simulink model "dec_consensus_dead"  (R2022b)
settings: Solver=FixedStepAuto  StartTime=0.0  StopTime=tf  FixedStep=dt  RelTol=1e-3
values from neighbouring files (symbols this model uses):
  A_an_n2 = ss_An.A    [squared_formation_dec.m]
  A_an_n3 = ss_An.A    [squared_formation_dec.m]
  A_an_n4 = ss_An.A    [squared_formation_dec.m]
  A_an_n6 = ss_An.A    [squared_formation_dec.m]
  alpha = binvar(nt,nr)    [main_red_based_TA.m]    (also in motivating_ex_four.m = 25; old_red_based_TA.m = binvar(nt*nr,1); red_consensus.m = 50; red_consensus_2D.m = 50)
  B = eye(n)    [red_consensus.m]    (also in red_consensus_2D.m = eye(2*n); rendez_vous.m = eye(2*n_t3); squared_formation.m = eye(2*n_t2); squared_formation_dec.m = eye(2*n_t2))
  B_an_n2 = ss_An.B    [squared_formation_dec.m]
  B_an_n3 = ss_An.B    [squared_formation_dec.m]
  B_an_n4 = ss_An.B    [squared_formation_dec.m]
  B_an_n6 = ss_An.B    [squared_formation_dec.m]
  C_an_n2 = ss_An.C    [squared_formation_dec.m]
  C_an_n3 = ss_An.C    [squared_formation_dec.m]
  C_an_n4 = ss_An.C    [squared_formation_dec.m]
  C_an_n6 = ss_An.C    [squared_formation_dec.m]
  C_n2 = blkdiag(L_n2,L_n2)    [squared_formation_dec.m]
  C_n3 = blkdiag(L_n3,L_n3)    [squared_formation_dec.m]
  C_n4 = blkdiag(L_n4,L_n4)    [squared_formation_dec.m]
  C_n6 = blkdiag(L_n6,L_n6)    [squared_formation_dec.m]
  C_opt = 1    [motivating_ex_four.m]    (also in red_consensus.m; red_consensus_2D.m = eye(2); rendez_vous.m = eye(2); squared_formation.m = eye(2))
  D_an_n2 = ss_An.D    [squared_formation_dec.m]
  D_an_n3 = ss_An.D    [squared_formation_dec.m]
  D_an_n4 = ss_An.D    [squared_formation_dec.m]
  D_an_n6 = ss_An.D    [squared_formation_dec.m]
  delta_n2 = [delta_x_t2(Idx2);delta_y_t2(Idx2)]    [squared_formation_dec.m]
  delta_n3 = [delta_x_t2(Idx3);delta_y_t2(Idx3)]    [squared_formation_dec.m]
  delta_n4 = [delta_x_t2(Idx4);delta_y_t2(Idx4)]    [squared_formation_dec.m]
  delta_n6 = [delta_x_t2(Idx6);delta_y_t2(Idx6)]    [squared_formation_dec.m]
  f = 0.2    [consensus.m]    (also in consensus_sat.m; red_consensus.m = 1; red_consensus_2D.m; rendez_vous.m)
  sig_vec = ones(num,1)    [rendez_vous.m]    (also in squared_formation.m; squared_formation_dec.m; triangular_formation.m)
  th = 0.05    [motivating_ex_four.m]    (also in red_consensus.m; red_consensus_2D.m; triangular_formation.m)
  u_max_n2 = [u_max1;u_max2;u_max3]    [motivating_ex_four.m]    (also in squared_formation_dec.m = [u_max_x(idx_n2);u_max_y(idx_n2)])
  u_max_n3 = [u_max2;u_max3;u_max4]    [motivating_ex_four.m]    (also in squared_formation_dec.m = [u_max_x(idx_n3);u_max_y(idx_n3)])
  u_max_n4 = [u_max3;u_max4]    [motivating_ex_four.m]    (also in squared_formation_dec.m = [u_max_x(idx_n4);u_max_y(idx_n4)])
  u_max_n6 = [u_max_x(idx_n6);u_max_y(idx_n6)]    [squared_formation_dec.m]
  W_an0_n2 = dcgain(W_an)    [squared_formation_dec.m]
  W_an0_n3 = dcgain(W_an)    [squared_formation_dec.m]
  W_an0_n4 = dcgain(W_an)    [squared_formation_dec.m]
  W_an0_n6 = dcgain(W_an)    [squared_formation_dec.m]
  x0_n2 = x0_cc2(Idx2)    [squared_formation_dec.m]
  x0_n3 = x0_cc2(Idx3)    [squared_formation_dec.m]
  x0_n4 = x0_cc2(Idx4)    [squared_formation_dec.m]
  x0_n6 = x0_cc2(Idx6)    [squared_formation_dec.m]
  x_an0 = zeros(max(size(A_an)),1)    [red_consensus.m]    (also in red_consensus_2D.m; rendez_vous.m; squared_formation.m; squared_formation_dec.m = zeros(max(size(A_an_n2)),1))
  x_opt0 = 0    [red_consensus.m]    (also in red_consensus_2D.m = zeros(2,1); rendez_vous.m = zeros(2,1); squared_formation.m = zeros(2,1); squared_formation_dec.m = zeros(2,1))
  y0_n2 = y0_cc2(Idx2)    [squared_formation_dec.m]
  y0_n3 = y0_cc2(Idx3)    [squared_formation_dec.m]
  y0_n4 = y0_cc2(Idx4)    [squared_formation_dec.m]
  y0_n6 = y0_cc2(Idx6)    [squared_formation_dec.m]
settings Model: Creator=lorenzo  LastModifiedBy=lorenzo
settings SolverCC: ZeroCrossControl=DisableAll
settings OptimizationCC: ReuseModelBlockBuffer=on
settings DebuggingCC: IgnoredZcDiagnostic=none

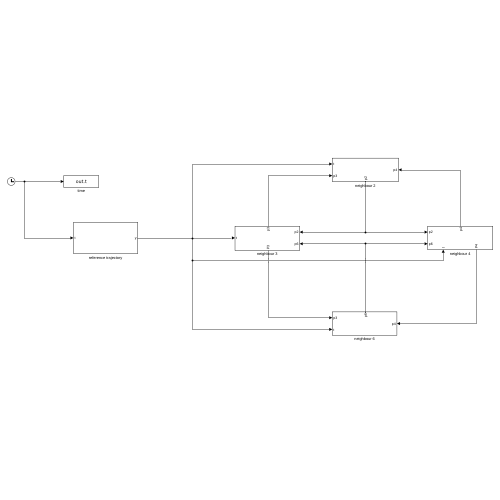
[thumbnail: Simulink's stored preview of the top-level diagram]
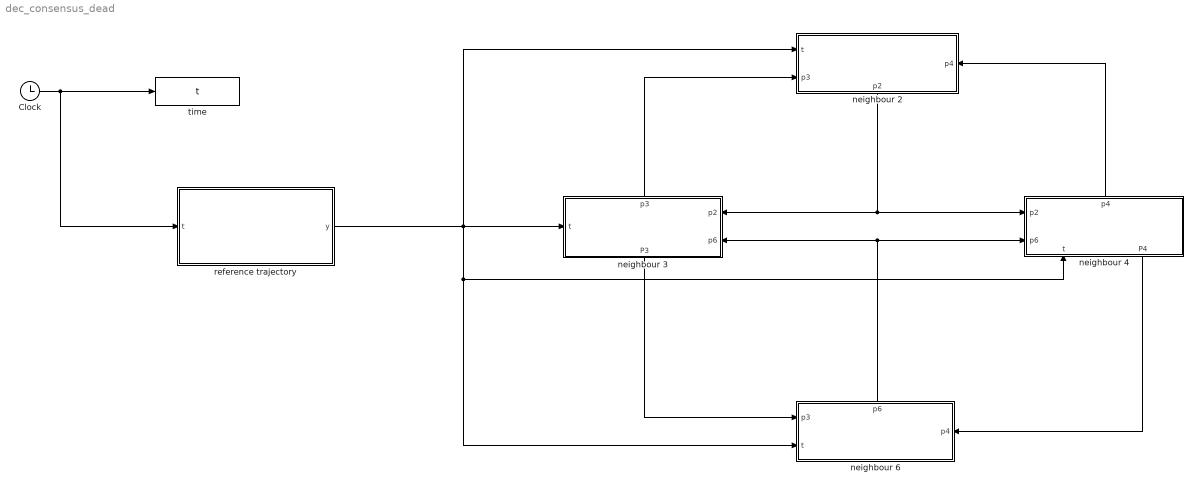
== system dec_consensus_dead ==
  Clock : Clock
  neighbour 2 : Subsystem
      settings: PortSchema="{\"entries\":[{\"content\":{\"sides\":[{\"content\":{\"connectorIds\":[\"In1\",\"In2\"]},\"type\":\"ConnectorPlacement.EquallySpacedRectSide\",\"uuid\":\"42d45d69-a067-4c4a-b460-9645b2520483\"},{\"content\":{\"connectorIds\":[\"In3\"],\"side\":\"RIGHT\"},\"type\":\"ConnectorPlacement.EquallySpacedRectSide\",\"uuid\":\"53118285-a7d6-411a-9657-0b0e62d2f91b\"},{\"content\":{\"side\":\"TOP\"},\"type\":\"ConnectorPlacement.EquallySpacedRectSide\",\"uuid\":\"c5fddcba-64f0-463e-bedc-85532df37ac6\"},{\"content\":{\"connectorIds\":[\"Out1\"],\"side\":\"BOTTOM\"},\"type\":\"ConnectorPlacement.EquallySpacedRectSide\",\"uuid\":\"9dd71ffb-fb5e-44d1-a551-03308aeb134d\"}]},\"type\":\"ConnectorPlacement.EquallySpacedConnector\",\"uuid\":\"f4aceda7-89b5-4913-ba88-086eac968990\"}],\"packageUris\":[\"http://schema.mathworks.com/mf0/Connector/R2020b\"],\"version\":\"1.0\"}"
  neighbour 3 : Subsystem
      settings: PortSchema="{\"entries\":[{\"content\":{\"sides\":[{\"content\":{\"connectorIds\":[\"In1\"]},\"type\":\"ConnectorPlacement.EquallySpacedRectSide\",\"uuid\":\"412d90c3-89ad-4a26-a7b4-17fcb9c5df26\"},{\"content\":{\"connectorIds\":[\"In2\",\"In3\"],\"side\":\"RIGHT\"},\"type\":\"ConnectorPlacement.EquallySpacedRectSide\",\"uuid\":\"01a5af2d-3d53-416a-b9d5-630e143a8097\"},{\"content\":{\"connectorIds\":[\"Out2\"],\"side\":\"TOP\"},\"type\":\"ConnectorPlacement.EquallySpacedRectSide\",\"uuid\":\"85dc40f1-eb1d-4853-882a-9bc97db5a7e5\"},{\"content\":{\"connectorIds\":[\"Out1\"],\"side\":\"BOTTOM\"},\"type\":\"ConnectorPlacement.EquallySpacedRectSide\",\"uuid\":\"c34b30fc-08ec-45f3-a893-1f001698b950\"}]},\"type\":\"ConnectorPlacement.EquallySpacedConnector\",\"uuid\":\"911331bd-e576-4dd9-be2f-03629677e448\"}],\"packageUris\":[\"http://schema.mathworks.com/mf0/Connector/R2020b\"],\"version\":\"1.0\"}"
  neighbour 4 : Subsystem
      settings: PortSchema="{\"entries\":[{\"content\":{\"sides\":[{\"content\":{\"connectorIds\":[\"In1\",\"In2\"]},\"type\":\"ConnectorPlacement.EquallySpacedRectSide\",\"uuid\":\"412d90c3-89ad-4a26-a7b4-17fcb9c5df26\"},{\"content\":{\"side\":\"RIGHT\"},\"type\":\"ConnectorPlacement.EquallySpacedRectSide\",\"uuid\":\"01a5af2d-3d53-416a-b9d5-630e143a8097\"},{\"content\":{\"connectorIds\":[\"Out2\"],\"side\":\"TOP\"},\"type\":\"ConnectorPlacement.EquallySpacedRectSide\",\"uuid\":\"85dc40f1-eb1d-4853-882a-9bc97db5a7e5\"},{\"content\":{\"connectorIds\":[\"In3\",\"Out1\"],\"side\":\"BOTTOM\"},\"type\":\"ConnectorPlacement.EquallySpacedRectSide\",\"uuid\":\"9a5a81a9-9beb-46ec-908b-79f317a66083\"}]},\"type\":\"ConnectorPlacement.EquallySpacedConnector\",\"uuid\":\"911331bd-e576-4dd9-be2f-03629677e448\"}],\"packageUris\":[\"http://schema.mathworks.com/mf0/Connector/R2020b\"],\"version\":\"1.0\"}"
  neighbour 6 : Subsystem
      settings: PortSchema="{\"entries\":[{\"content\":{\"sides\":[{\"content\":{\"connectorIds\":[\"In1\",\"In2\"]},\"type\":\"ConnectorPlacement.EquallySpacedRectSide\",\"uuid\":\"42d45d69-a067-4c4a-b460-9645b2520483\"},{\"content\":{\"connectorIds\":[\"In3\"],\"side\":\"RIGHT\"},\"type\":\"ConnectorPlacement.EquallySpacedRectSide\",\"uuid\":\"53118285-a7d6-411a-9657-0b0e62d2f91b\"},{\"content\":{\"connectorIds\":[\"Out1\"],\"side\":\"TOP\"},\"type\":\"ConnectorPlacement.EquallySpacedRectSide\",\"uuid\":\"c5fddcba-64f0-463e-bedc-85532df37ac6\"}]},\"type\":\"ConnectorPlacement.EquallySpacedConnector\",\"uuid\":\"f4aceda7-89b5-4913-ba88-086eac968990\"}],\"packageUris\":[\"http://schema.mathworks.com/mf0/Connector/R2020b\"],\"version\":\"1.0\"}"
  reference trajectory : Subsystem
  time : ToWorkspace  VariableName=t  SampleTime=-1
  wires:
  Clock/1 -> reference trajectory/1(t), time/1
  reference trajectory/1(y) -> neighbour 3/1(t), neighbour 6/2(t), neighbour 4/3(t), neighbour 2/1(t)
  neighbour 3/1(P3) -> neighbour 6/1(p3)
  neighbour 4/1(P4) -> neighbour 6/3(p4)
  neighbour 6/1(p6) -> neighbour 3/3(p6), neighbour 4/2(p6)
  neighbour 3/2(p3) -> neighbour 2/2(p3)
  neighbour 4/2(p4) -> neighbour 2/3(p4)
  neighbour 2/1(p2) -> neighbour 4/1(p2), neighbour 3/2(p2)

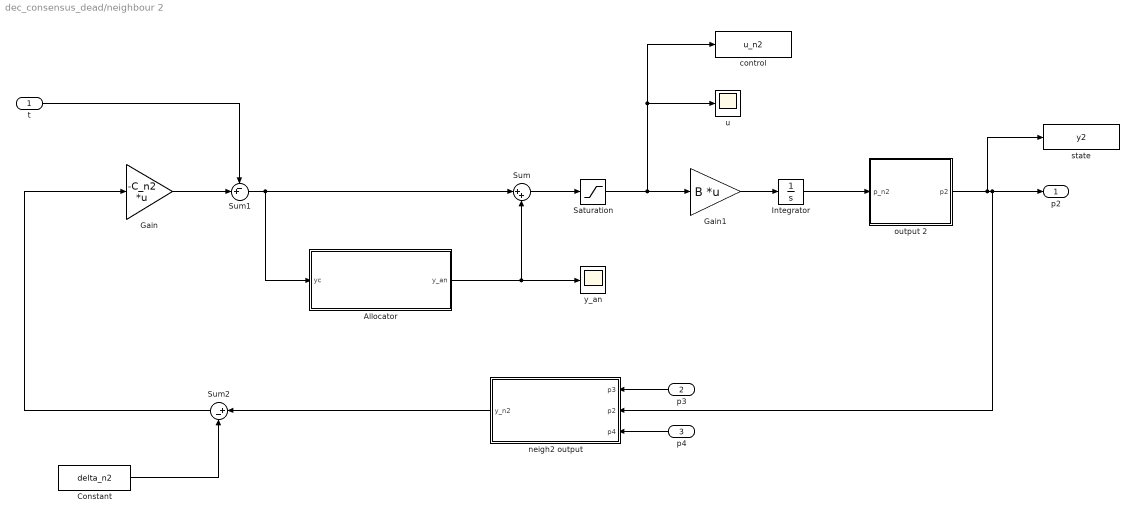
== system dec_consensus_dead/neighbour 2 ==
  t : Inport
  p3 : Inport  Port=2
  p4 : Inport  Port=3
  Allocator : Subsystem
  Constant : Constant  Value=delta_n2  VectorParams1D=off
  Gain : Gain  Gain=-C_n2  Multiplication=Matrix(K*u)
  Gain1 : Gain  Gain=B  Multiplication=Matrix(K*u)
  Integrator : Integrator  InitialCondition=[x0_n2;y0_n2]
  Saturation : Saturate  UpperLimit=u_max_n2  LowerLimit=-u_max_n2
  Sum : Sum  Inputs=|++
  Sum1 : Sum  Inputs=-+|  InputSameDT=on
  Sum2 : Sum  Inputs=|+-
  control : ToWorkspace  VariableName=u_n2  SampleTime=-1
  neigh2 output : MATLAB Function  TreatAsAtomicUnit=on
  output 2 : MATLAB Function  TreatAsAtomicUnit=on
  state : ToWorkspace  VariableName=y2  SampleTime=-1
  u : Scope
  y_an : Scope
  p2 : Outport
  wires:
  Constant/1 -> Sum2/2
  Allocator/1(y_an) -> Sum/2, y_an/1
  Gain1/1 -> Integrator/1
  Sum2/1 -> Gain/1
  Sum1/1 -> Allocator/1(yc), Sum/1
  Sum/1 -> Saturation/1
  Gain/1 -> Sum1/2
  t/1 -> Sum1/1
  Saturation/1 -> control/1, u/1, Gain1/1
  Integrator/1 -> output 2/1(p_n2)
  neigh2 output/1(y_n2) -> Sum2/1
  p3/1 -> neigh2 output/1(p3)
  p4/1 -> neigh2 output/3(p4)
  output 2/1(p2) -> state/1, neigh2 output/2(p2), p2/1

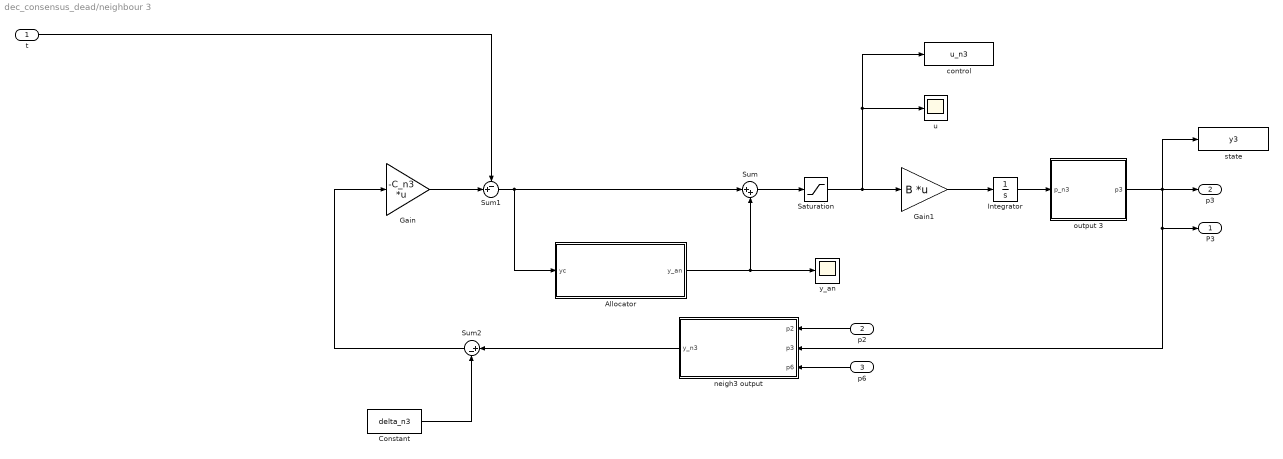
== system dec_consensus_dead/neighbour 3 ==
  t : Inport
  p2 : Inport  Port=2
  p6 : Inport  Port=3
  Allocator : Subsystem
  Constant : Constant  Value=delta_n3  VectorParams1D=off
  Gain : Gain  Gain=-C_n3  Multiplication=Matrix(K*u)
  Gain1 : Gain  Gain=B  Multiplication=Matrix(K*u)
  Integrator : Integrator  InitialCondition=[x0_n3;y0_n3]
  Saturation : Saturate  UpperLimit=u_max_n3  LowerLimit=-u_max_n3
  Sum : Sum  Inputs=|++
  Sum1 : Sum  Inputs=-+|  InputSameDT=on
  Sum2 : Sum  Inputs=|+-
  control : ToWorkspace  VariableName=u_n3  SampleTime=-1
  neigh3 output : MATLAB Function  TreatAsAtomicUnit=on
  output 3 : MATLAB Function  TreatAsAtomicUnit=on
  state : ToWorkspace  VariableName=y3  SampleTime=-1
  u : Scope
  y_an : Scope
  P3 : Outport
  p3 : Outport  Port=2
  wires:
  Constant/1 -> Sum2/2
  Allocator/1(y_an) -> Sum/2, y_an/1
  Gain1/1 -> Integrator/1
  Sum2/1 -> Gain/1
  Sum1/1 -> Allocator/1(yc), Sum/1
  Sum/1 -> Saturation/1
  Gain/1 -> Sum1/2
  t/1 -> Sum1/1
  Saturation/1 -> control/1, u/1, Gain1/1
  Integrator/1 -> output 3/1(p_n3)
  neigh3 output/1(y_n3) -> Sum2/1
  p2/1 -> neigh3 output/1(p2)
  p6/1 -> neigh3 output/3(p6)
  output 3/1(p3) -> state/1, neigh3 output/2(p3), P3/1, p3/1

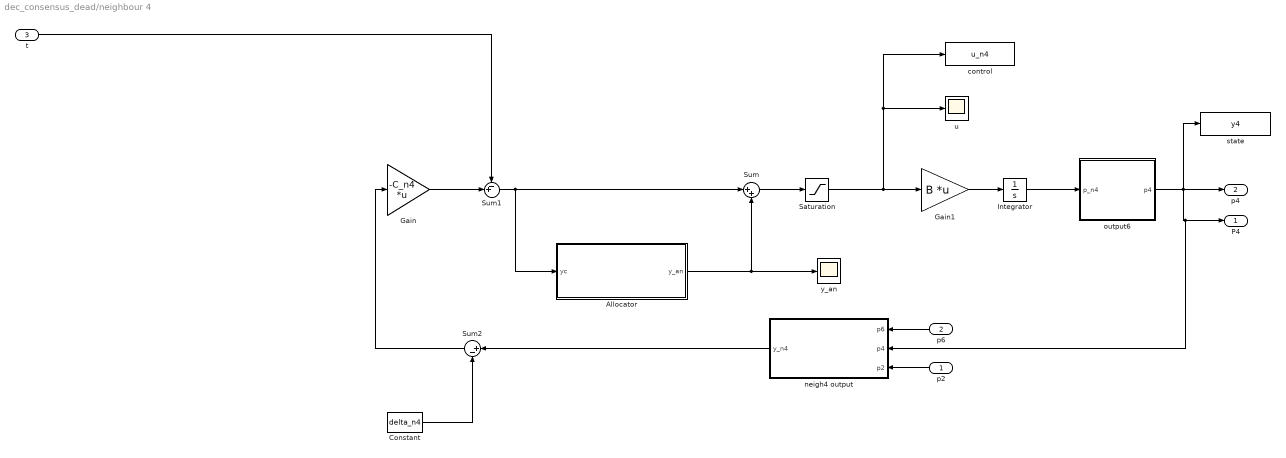
== system dec_consensus_dead/neighbour 4 ==
  p2 : Inport
  p6 : Inport  Port=2
  t : Inport  Port=3
  Allocator : Subsystem
  Constant : Constant  Value=delta_n4  VectorParams1D=off
  Gain : Gain  Gain=-C_n4  Multiplication=Matrix(K*u)
  Gain1 : Gain  Gain=B  Multiplication=Matrix(K*u)
  Integrator : Integrator  InitialCondition=[x0_n4;y0_n4]
  Saturation : Saturate  UpperLimit=u_max_n4  LowerLimit=-u_max_n4
  Sum : Sum  Inputs=|++
  Sum1 : Sum  Inputs=-+|  InputSameDT=on
  Sum2 : Sum  Inputs=|+-
  control : ToWorkspace  VariableName=u_n4  SampleTime=-1
  neigh4 output : MATLAB Function  TreatAsAtomicUnit=on
  output6 : MATLAB Function  TreatAsAtomicUnit=on
  state : ToWorkspace  VariableName=y4  SampleTime=-1
  u : Scope
  y_an : Scope
  P4 : Outport
  p4 : Outport  Port=2
  wires:
  Constant/1 -> Sum2/2
  Allocator/1(y_an) -> Sum/2, y_an/1
  Gain1/1 -> Integrator/1
  Sum2/1 -> Gain/1
  Sum1/1 -> Allocator/1(yc), Sum/1
  Sum/1 -> Saturation/1
  Gain/1 -> Sum1/2
  t/1 -> Sum1/1
  Saturation/1 -> control/1, u/1, Gain1/1
  Integrator/1 -> output6/1(p_n4)
  neigh4 output/1(y_n4) -> Sum2/1
  p2/1 -> neigh4 output/3(p2)
  p6/1 -> neigh4 output/1(p6)
  output6/1(p4) -> state/1, neigh4 output/2(p4), P4/1, p4/1

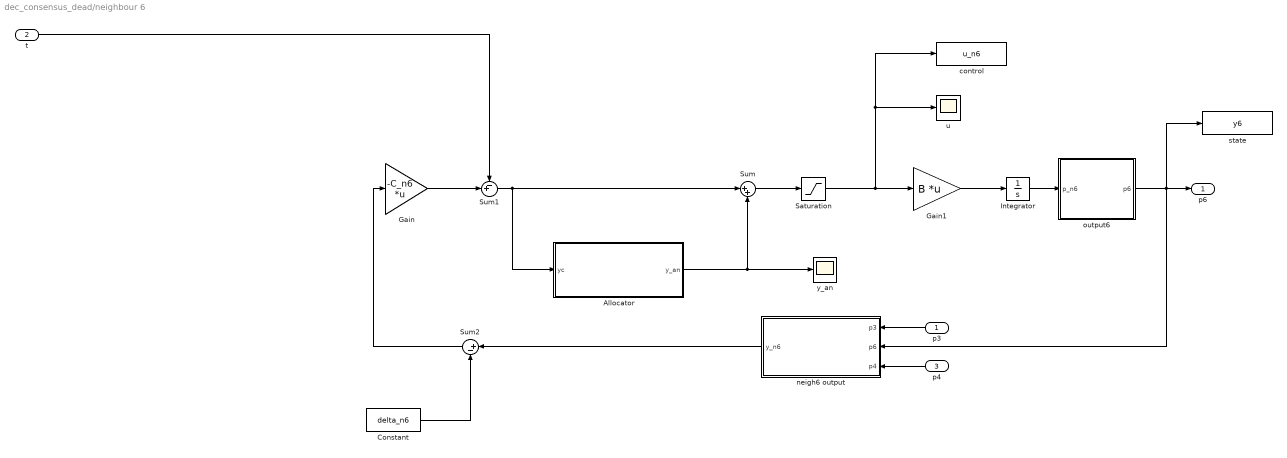
== system dec_consensus_dead/neighbour 6 ==
  p3 : Inport
  t : Inport  Port=2
  p4 : Inport  Port=3
  Allocator : Subsystem
  Constant : Constant  Value=delta_n6  VectorParams1D=off
  Gain : Gain  Gain=-C_n6  Multiplication=Matrix(K*u)
  Gain1 : Gain  Gain=B  Multiplication=Matrix(K*u)
  Integrator : Integrator  InitialCondition=[x0_n6;y0_n6]
  Saturation : Saturate  UpperLimit=u_max_n6  LowerLimit=-u_max_n6
  Sum : Sum  Inputs=|++
  Sum1 : Sum  Inputs=-+|  InputSameDT=on
  Sum2 : Sum  Inputs=|+-
  control : ToWorkspace  VariableName=u_n6  SampleTime=-1
  neigh6 output : MATLAB Function  TreatAsAtomicUnit=on
  output6 : MATLAB Function  TreatAsAtomicUnit=on
  state : ToWorkspace  VariableName=y6  SampleTime=-1
  u : Scope
  y_an : Scope
  p6 : Outport
  wires:
  Constant/1 -> Sum2/2
  Allocator/1(y_an) -> Sum/2, y_an/1
  Gain1/1 -> Integrator/1
  Sum2/1 -> Gain/1
  Sum1/1 -> Allocator/1(yc), Sum/1
  Sum/1 -> Saturation/1
  Gain/1 -> Sum1/2
  t/1 -> Sum1/1
  Saturation/1 -> control/1, u/1, Gain1/1
  Integrator/1 -> output6/1(p_n6)
  output6/1(p6) -> state/1, neigh6 output/2(p6), p6/1
  neigh6 output/1(y_n6) -> Sum2/1
  p3/1 -> neigh6 output/1(p3)
  p4/1 -> neigh6 output/3(p4)

== system dec_consensus_dead/reference trajectory ==
  t : Inport
  Constant1 : Constant  Value=sig_vec  VectorParams1D=off
  Constant2 : Constant  Value=sig_vec  VectorParams1D=off
  MATLAB Function : MATLAB Function  TreatAsAtomicUnit=on
  Product : Product
  Product1 : Product
  Sine Wave Function : Sin  TimeSource=Use external signal  Frequency=f  SampleTime=0
  Sine Wave Function1 : Sin  TimeSource=Use external signal  Frequency=f  Phase=pi/2  SampleTime=0
  y : Outport
  wires:
  Sine Wave Function1/1 -> Product1/1
  Sine Wave Function/1 -> Product/1
  Constant2/1 -> Product1/2
  Product/1 -> MATLAB Function/2(seno)
  Constant1/1 -> Product/2
  Product1/1 -> MATLAB Function/1(coseno)
  t/1 -> Sine Wave Function1/1, Sine Wave Function/1
  MATLAB Function/1(y) -> y/1

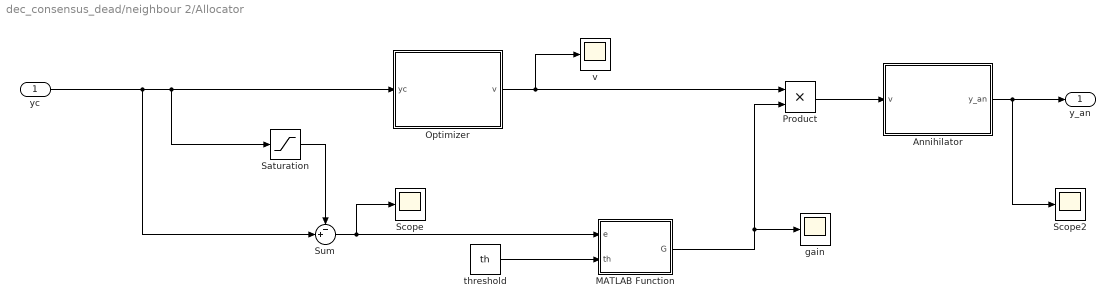
== system dec_consensus_dead/neighbour 2/Allocator ==
  yc : Inport
  Annihilator : Subsystem
  MATLAB Function : MATLAB Function  TreatAsAtomicUnit=on
  Optimizer : Subsystem
  Product : Product
  Saturation : Saturate  UpperLimit=u_max_n2  LowerLimit=-u_max_n2
  Scope : Scope
  Scope2 : Scope
  Sum : Sum  Inputs=-+|
  gain : Scope
  threshold : Constant  Value=th
  v : Scope
  y_an : Outport
  wires:
  threshold/1 -> MATLAB Function/2(th)
  yc/1 -> Sum/2, Saturation/1, Optimizer/1(yc)
  Product/1 -> Annihilator/1(v)
  Annihilator/1(y_an) -> Scope2/1, y_an/1
  MATLAB Function/1(G) -> Product/2, gain/1
  Optimizer/1(v) -> v/1, Product/1
  Saturation/1 -> Sum/1
  Sum/1 -> MATLAB Function/1(e), Scope/1

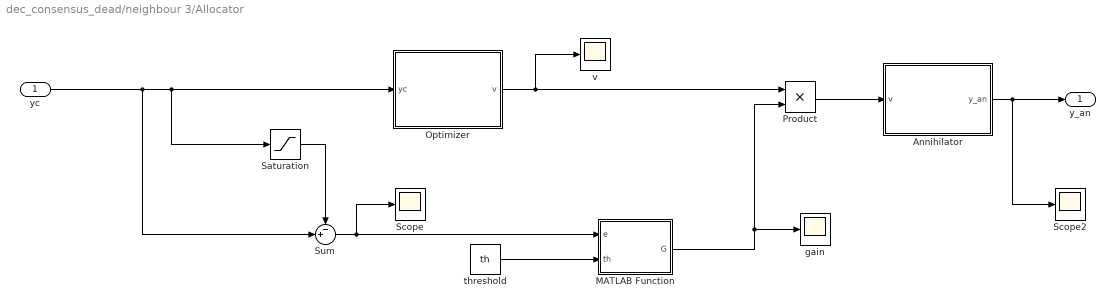
== system dec_consensus_dead/neighbour 3/Allocator ==
  yc : Inport
  Annihilator : Subsystem
  MATLAB Function : MATLAB Function  TreatAsAtomicUnit=on
  Optimizer : Subsystem
  Product : Product
  Saturation : Saturate  UpperLimit=u_max_n3  LowerLimit=-u_max_n3
  Scope : Scope
  Scope2 : Scope
  Sum : Sum  Inputs=-+|
  gain : Scope
  threshold : Constant  Value=th
  v : Scope
  y_an : Outport
  wires:
  threshold/1 -> MATLAB Function/2(th)
  yc/1 -> Sum/2, Saturation/1, Optimizer/1(yc)
  Product/1 -> Annihilator/1(v)
  Annihilator/1(y_an) -> Scope2/1, y_an/1
  MATLAB Function/1(G) -> Product/2, gain/1
  Optimizer/1(v) -> v/1, Product/1
  Saturation/1 -> Sum/1
  Sum/1 -> MATLAB Function/1(e), Scope/1

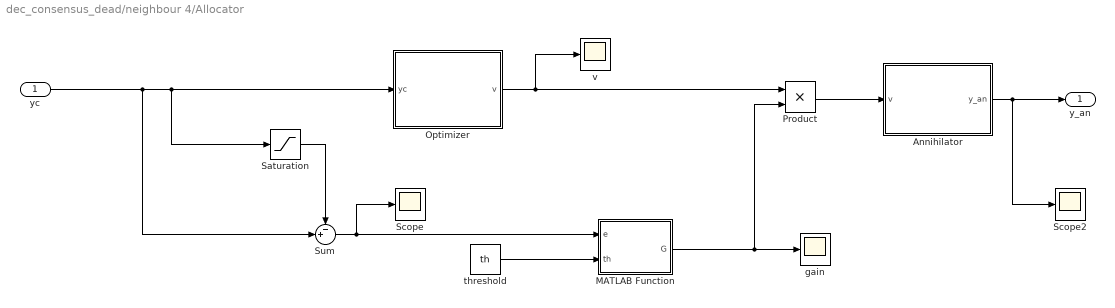
== system dec_consensus_dead/neighbour 4/Allocator ==
  yc : Inport
  Annihilator : Subsystem
  MATLAB Function : MATLAB Function  TreatAsAtomicUnit=on
  Optimizer : Subsystem
  Product : Product
  Saturation : Saturate  UpperLimit=u_max_n4  LowerLimit=-u_max_n4
  Scope : Scope
  Scope2 : Scope
  Sum : Sum  Inputs=-+|
  gain : Scope
  threshold : Constant  Value=th
  v : Scope
  y_an : Outport
  wires:
  threshold/1 -> MATLAB Function/2(th)
  yc/1 -> Sum/2, Saturation/1, Optimizer/1(yc)
  Product/1 -> Annihilator/1(v)
  Annihilator/1(y_an) -> Scope2/1, y_an/1
  MATLAB Function/1(G) -> Product/2, gain/1
  Optimizer/1(v) -> v/1, Product/1
  Saturation/1 -> Sum/1
  Sum/1 -> MATLAB Function/1(e), Scope/1

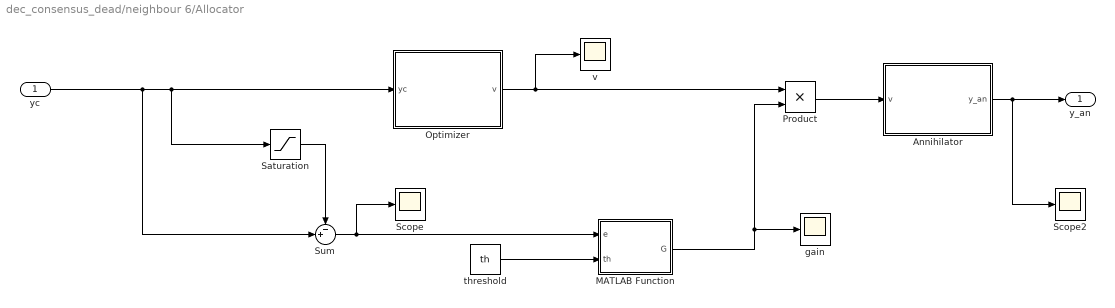
== system dec_consensus_dead/neighbour 6/Allocator ==
  yc : Inport
  Annihilator : Subsystem
  MATLAB Function : MATLAB Function  TreatAsAtomicUnit=on
  Optimizer : Subsystem
  Product : Product
  Saturation : Saturate  UpperLimit=u_max_n6  LowerLimit=-u_max_n6
  Scope : Scope
  Scope2 : Scope
  Sum : Sum  Inputs=-+|
  gain : Scope
  threshold : Constant  Value=th
  v : Scope
  y_an : Outport
  wires:
  threshold/1 -> MATLAB Function/2(th)
  yc/1 -> Sum/2, Saturation/1, Optimizer/1(yc)
  Product/1 -> Annihilator/1(v)
  Annihilator/1(y_an) -> Scope2/1, y_an/1
  MATLAB Function/1(G) -> Product/2, gain/1
  Optimizer/1(v) -> v/1, Product/1
  Saturation/1 -> Sum/1
  Sum/1 -> MATLAB Function/1(e), Scope/1

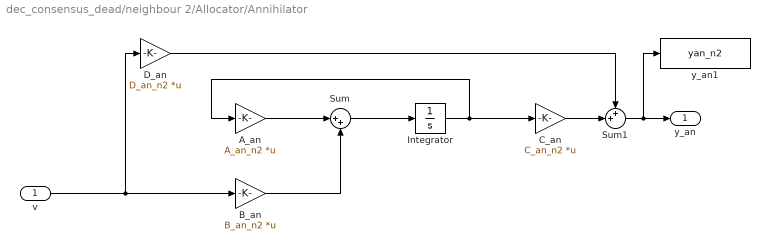
== system dec_consensus_dead/neighbour 2/Allocator/Annihilator ==
  v : Inport
  A_an : Gain  Gain=A_an_n2  Multiplication=Matrix(K*u) (u vector)
  B_an : Gain  Gain=B_an_n2  Multiplication=Matrix(K*u) (u vector)
  C_an : Gain  Gain=C_an_n2  Multiplication=Matrix(K*u) (u vector)
  D_an : Gain  Gain=D_an_n2  Multiplication=Matrix(K*u) (u vector)
  Integrator : Integrator  InitialCondition=x_an0
  Sum : Sum  Inputs=|++
  Sum1 : Sum  Inputs=++|
  y_an1 : ToWorkspace  VariableName=yan_n2  SampleTime=-1
  y_an : Outport
  wires:
  Integrator/1 -> C_an/1, A_an/1
  B_an/1 -> Sum/2
  A_an/1 -> Sum/1
  Sum/1 -> Integrator/1
  C_an/1 -> Sum1/2
  D_an/1 -> Sum1/1
  Sum1/1 -> y_an1/1, y_an/1
  v/1 -> B_an/1, D_an/1

== system dec_consensus_dead/neighbour 2/Allocator/Optimizer ==
  yc : Inport
  C_opt : Gain  Gain=C_opt  Multiplication=Matrix(K*u) (u vector)
  C_opt1 : Constant  Value=C_opt
  Constant : Constant  Value=alpha
  Integrator : Integrator  InitialCondition=x_opt0
  Wan0 : Constant  Value=W_an0_n2  VectorParams1D=off
  dx_opt : MATLAB Function  TreatAsAtomicUnit=on
  u_max : Constant  Value=u_max_n2
  v : Outport
  wires:
  Integrator/1 -> C_opt/1, dx_opt/4(x_opt)
  dx_opt/1(dx_opt) -> Integrator/1
  C_opt/1 -> v/1
  Constant/1 -> dx_opt/1(alpha)
  yc/1 -> dx_opt/2(yc)
  Wan0/1 -> dx_opt/3(Wan0)
  u_max/1 -> dx_opt/5(u_max)
  C_opt1/1 -> dx_opt/6(C_opt)

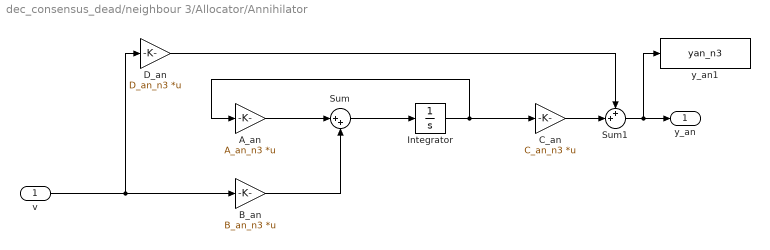
== system dec_consensus_dead/neighbour 3/Allocator/Annihilator ==
  v : Inport
  A_an : Gain  Gain=A_an_n3  Multiplication=Matrix(K*u) (u vector)
  B_an : Gain  Gain=B_an_n3  Multiplication=Matrix(K*u) (u vector)
  C_an : Gain  Gain=C_an_n3  Multiplication=Matrix(K*u) (u vector)
  D_an : Gain  Gain=D_an_n3  Multiplication=Matrix(K*u) (u vector)
  Integrator : Integrator  InitialCondition=x_an0
  Sum : Sum  Inputs=|++
  Sum1 : Sum  Inputs=++|
  y_an1 : ToWorkspace  VariableName=yan_n3  SampleTime=-1
  y_an : Outport
  wires:
  Integrator/1 -> C_an/1, A_an/1
  B_an/1 -> Sum/2
  A_an/1 -> Sum/1
  Sum/1 -> Integrator/1
  C_an/1 -> Sum1/2
  D_an/1 -> Sum1/1
  Sum1/1 -> y_an1/1, y_an/1
  v/1 -> B_an/1, D_an/1

== system dec_consensus_dead/neighbour 3/Allocator/Optimizer ==
  yc : Inport
  C_opt : Gain  Gain=C_opt  Multiplication=Matrix(K*u) (u vector)
  C_opt1 : Constant  Value=C_opt
  Constant : Constant  Value=alpha
  Integrator : Integrator  InitialCondition=x_opt0
  Wan0 : Constant  Value=W_an0_n3  VectorParams1D=off
  dx_opt : MATLAB Function  TreatAsAtomicUnit=on
  u_max : Constant  Value=u_max_n3
  v : Outport
  wires:
  Integrator/1 -> C_opt/1, dx_opt/4(x_opt)
  dx_opt/1(dx_opt) -> Integrator/1
  C_opt/1 -> v/1
  Constant/1 -> dx_opt/1(alpha)
  yc/1 -> dx_opt/2(yc)
  Wan0/1 -> dx_opt/3(Wan0)
  u_max/1 -> dx_opt/5(u_max)
  C_opt1/1 -> dx_opt/6(C_opt)

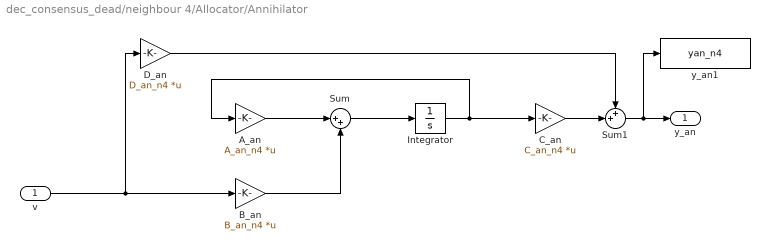
== system dec_consensus_dead/neighbour 4/Allocator/Annihilator ==
  v : Inport
  A_an : Gain  Gain=A_an_n4  Multiplication=Matrix(K*u) (u vector)
  B_an : Gain  Gain=B_an_n4  Multiplication=Matrix(K*u) (u vector)
  C_an : Gain  Gain=C_an_n4  Multiplication=Matrix(K*u) (u vector)
  D_an : Gain  Gain=D_an_n4  Multiplication=Matrix(K*u) (u vector)
  Integrator : Integrator  InitialCondition=x_an0
  Sum : Sum  Inputs=|++
  Sum1 : Sum  Inputs=++|
  y_an1 : ToWorkspace  VariableName=yan_n4  SampleTime=-1
  y_an : Outport
  wires:
  Integrator/1 -> C_an/1, A_an/1
  B_an/1 -> Sum/2
  A_an/1 -> Sum/1
  Sum/1 -> Integrator/1
  C_an/1 -> Sum1/2
  D_an/1 -> Sum1/1
  Sum1/1 -> y_an1/1, y_an/1
  v/1 -> B_an/1, D_an/1

== system dec_consensus_dead/neighbour 4/Allocator/Optimizer ==
  yc : Inport
  C_opt : Gain  Gain=C_opt  Multiplication=Matrix(K*u) (u vector)
  C_opt1 : Constant  Value=C_opt
  Constant : Constant  Value=alpha
  Integrator : Integrator  InitialCondition=x_opt0
  Wan0 : Constant  Value=W_an0_n4  VectorParams1D=off
  dx_opt : MATLAB Function  TreatAsAtomicUnit=on
  u_max : Constant  Value=u_max_n4
  v : Outport
  wires:
  Integrator/1 -> C_opt/1, dx_opt/4(x_opt)
  dx_opt/1(dx_opt) -> Integrator/1
  C_opt/1 -> v/1
  Constant/1 -> dx_opt/1(alpha)
  yc/1 -> dx_opt/2(yc)
  Wan0/1 -> dx_opt/3(Wan0)
  u_max/1 -> dx_opt/5(u_max)
  C_opt1/1 -> dx_opt/6(C_opt)

== system dec_consensus_dead/neighbour 6/Allocator/Annihilator ==
  v : Inport
  A_an : Gain  Gain=A_an_n6  Multiplication=Matrix(K*u) (u vector)
  B_an : Gain  Gain=B_an_n6  Multiplication=Matrix(K*u) (u vector)
  C_an : Gain  Gain=C_an_n6  Multiplication=Matrix(K*u) (u vector)
  D_an : Gain  Gain=D_an_n6  Multiplication=Matrix(K*u) (u vector)
  Integrator : Integrator  InitialCondition=x_an0
  Sum : Sum  Inputs=|++
  Sum1 : Sum  Inputs=++|
  y_an1 : ToWorkspace  VariableName=yan_n6  SampleTime=-1
  y_an : Outport
  wires:
  Integrator/1 -> C_an/1, A_an/1
  B_an/1 -> Sum/2
  A_an/1 -> Sum/1
  Sum/1 -> Integrator/1
  C_an/1 -> Sum1/2
  D_an/1 -> Sum1/1
  Sum1/1 -> y_an1/1, y_an/1
  v/1 -> B_an/1, D_an/1

== system dec_consensus_dead/neighbour 6/Allocator/Optimizer ==
  yc : Inport
  C_opt : Gain  Gain=C_opt  Multiplication=Matrix(K*u) (u vector)
  C_opt1 : Constant  Value=C_opt
  Constant : Constant  Value=alpha
  Integrator : Integrator  InitialCondition=x_opt0
  Wan0 : Constant  Value=W_an0_n6  VectorParams1D=off
  dx_opt : MATLAB Function  TreatAsAtomicUnit=on
  u_max : Constant  Value=u_max_n6
  v : Outport
  wires:
  Integrator/1 -> C_opt/1, dx_opt/4(x_opt)
  dx_opt/1(dx_opt) -> Integrator/1
  C_opt/1 -> v/1
  Constant/1 -> dx_opt/1(alpha)
  yc/1 -> dx_opt/2(yc)
  Wan0/1 -> dx_opt/3(Wan0)
  u_max/1 -> dx_opt/5(u_max)
  C_opt1/1 -> dx_opt/6(C_opt)

== matlab function dec_consensus_dead/neighbour 2/neigh2 output ==
  data: p3 input; y_n2 output; p2 input; p4 input
function y_n2 = fcn(p3,p2,p4)

y_n2 = [p3(1);p2(1);p4(1);p3(2);p2(2);p4(2)];

== matlab function dec_consensus_dead/neighbour 2/output 2 ==
  data: p_n2 input; p2 output
function p2 = fcn(p_n2)

p2 = [p_n2(2),p_n2(5)];

== matlab function dec_consensus_dead/neighbour 3/neigh3 output ==
  data: p2 input; p3 input; y_n3 output; p6 input
function y_n3 = fcn(p2,p3,p6)

y_n3 = [p2(1);p3(1);p6(1);p2(2);p3(2);p6(2)];

== matlab function dec_consensus_dead/neighbour 3/output 3 ==
  data: p_n3 input; p3 output
function p3 = fcn(p_n3)

p3 = [p_n3(2),p_n3(5)];

== matlab function dec_consensus_dead/neighbour 6/output6 ==
  data: p_n6 input; p6 output
function p6 = fcn(p_n6)

p6 = [p_n6(2),p_n6(5)];

== matlab function dec_consensus_dead/neighbour 6/neigh6 output ==
  data: p3 input; p6 input; p4 input; y_n6 output
function y_n6 = fcn(p3,p6,p4)

y_n6 = [p3(1);p6(1);p4(1);p3(2);p6(2);p4(2)];

== matlab function dec_consensus_dead/neighbour 4/neigh4 output ==
  data: p6 input; p4 input; p2 input; y_n4 output
function y_n4 = fcn(p6,p4,p2)

y_n4 = [p6(1);p4(1);p2(1);p6(2);p4(2);p2(2)];

== matlab function dec_consensus_dead/neighbour 4/output6 ==
  data: p_n4 input; p4 output
function p4 = fcn(p_n4)

p4 = [p_n4(2),p_n4(5)];

== matlab function dec_consensus_dead/neighbour 2/Allocator/MATLAB Function ==
  data: e input; G output; th input
function G = fcn(e,th)
norm(e);
eps = th/2;

G=1;

% if ( norm(e) < th-eps )
%     G = 0;
% end
% if ( norm(e) > th )
%     G = 1;
% end
% if ( norm(e) <= th && norm(e) >= th-eps )
%     G = -2*((norm(e)-(th-eps))/eps)^3+3*((norm(e)-(th-eps))/eps)^2;
% end

== matlab function dec_consensus_dead/reference trajectory/MATLAB Function ==
  data: coseno input; y output; seno input
function y = fcn(coseno, seno)

y = [coseno;seno];

== matlab function dec_consensus_dead/neighbour 6/Allocator/MATLAB Function ==
  data: e input; G output; th input
function G = fcn(e,th)
norm(e);
eps = th/2;

G=1;

% if ( norm(e) < th-eps )
%     G = 0;
% end
% if ( norm(e) > th )
%     G = 1;
% end
% if ( norm(e) <= th && norm(e) >= th-eps )
%     G = -2*((norm(e)-(th-eps))/eps)^3+3*((norm(e)-(th-eps))/eps)^2;
% end

== matlab function dec_consensus_dead/neighbour 2/Allocator/Optimizer/dx_opt ==
  data: dx_opt output; alpha input; yc input; Wan0 input; x_opt input; u_max input; C_opt input
function dx_opt = opt_dyn(alpha,yc,Wan0,x_opt,u_max,C_opt)

dim = max(size(u_max));

ss_u = yc+Wan0*C_opt*x_opt;

ss_sat = ss_u;

for i=1:dim
    if ( abs(ss_u(i))>= u_max(i) )
        ss_sat(i) = sign(ss_u(i))*u_max(i);
    end
end

par_der = zeros(dim,dim);

for i =1:dim
    par_der(i,i) = dsat(ss_u(i),u_max(i),0.01);
end

grad = (ss_u-ss_sat)'*(Wan0*C_opt-par_der*Wan0*C_opt);

dx_opt = -alpha*grad';

== matlab function dec_consensus_dead/neighbour 6/Allocator/Optimizer/dx_opt ==
  data: dx_opt output; alpha input; yc input; Wan0 input; x_opt input; u_max input; C_opt input
function dx_opt = opt_dyn(alpha,yc,Wan0,x_opt,u_max,C_opt)

dim = max(size(u_max));

ss_u = yc+Wan0*C_opt*x_opt;

ss_sat = ss_u;

for i=1:dim
    if ( abs(ss_u(i))>= u_max(i) )
        ss_sat(i) = sign(ss_u(i))*u_max(i);
    end
end

par_der = zeros(dim,dim);

for i =1:dim
    par_der(i,i) = dsat(ss_u(i),u_max(i),0.01);
end

grad = (ss_u-ss_sat)'*(Wan0*C_opt-par_der*Wan0*C_opt);

dx_opt = -alpha*grad';

== matlab function dec_consensus_dead/neighbour 3/Allocator/MATLAB Function ==
  data: e input; G output; th input
function G = fcn(e,th)
norm(e);
eps = th/2;

G=1;

% if ( norm(e) < th-eps )
%     G = 0;
% end
% if ( norm(e) > th )
%     G = 1;
% end
% if ( norm(e) <= th && norm(e) >= th-eps )
%     G = -2*((norm(e)-(th-eps))/eps)^3+3*((norm(e)-(th-eps))/eps)^2;
% end

== matlab function dec_consensus_dead/neighbour 3/Allocator/Optimizer/dx_opt ==
  data: dx_opt output; alpha input; yc input; Wan0 input; x_opt input; u_max input; C_opt input
function dx_opt = opt_dyn(alpha,yc,Wan0,x_opt,u_max,C_opt)

dim = max(size(u_max));

ss_u = yc+Wan0*C_opt*x_opt;

ss_sat = ss_u;

for i=1:dim
    if ( abs(ss_u(i))>= u_max(i) )
        ss_sat(i) = sign(ss_u(i))*u_max(i);
    end
end

par_der = zeros(dim,dim);

for i =1:dim
    par_der(i,i) = dsat(ss_u(i),u_max(i),0.01);
end

grad = (ss_u-ss_sat)'*(Wan0*C_opt-par_der*Wan0*C_opt);

dx_opt = -alpha*grad';

== matlab function dec_consensus_dead/neighbour 4/Allocator/MATLAB Function ==
  data: e input; G output; th input
function G = fcn(e,th)
norm(e);
eps = th/2;

G=1;

% if ( norm(e) < th-eps )
%     G = 0;
% end
% if ( norm(e) > th )
%     G = 1;
% end
% if ( norm(e) <= th && norm(e) >= th-eps )
%     G = -2*((norm(e)-(th-eps))/eps)^3+3*((norm(e)-(th-eps))/eps)^2;
% end

== matlab function dec_consensus_dead/neighbour 4/Allocator/Optimizer/dx_opt ==
  data: dx_opt output; alpha input; yc input; Wan0 input; x_opt input; u_max input; C_opt input
function dx_opt = opt_dyn(alpha,yc,Wan0,x_opt,u_max,C_opt)

dim = max(size(u_max));

ss_u = yc+Wan0*C_opt*x_opt;

ss_sat = ss_u;

for i=1:dim
    if ( abs(ss_u(i))>= u_max(i) )
        ss_sat(i) = sign(ss_u(i))*u_max(i);
    end
end

par_der = zeros(dim,dim);

for i =1:dim
    par_der(i,i) = dsat(ss_u(i),u_max(i),0.01);
end

grad = (ss_u-ss_sat)'*(Wan0*C_opt-par_der*Wan0*C_opt);

dx_opt = -alpha*grad';
